simulink model "HODB"  (R2018b)
settings: Solver=FixedStepAuto  StartTime=0.0  StopTime=25  FixedStep=0.0025  RelTol=1e-3
settings Model: Creator=User  LastModifiedBy=User

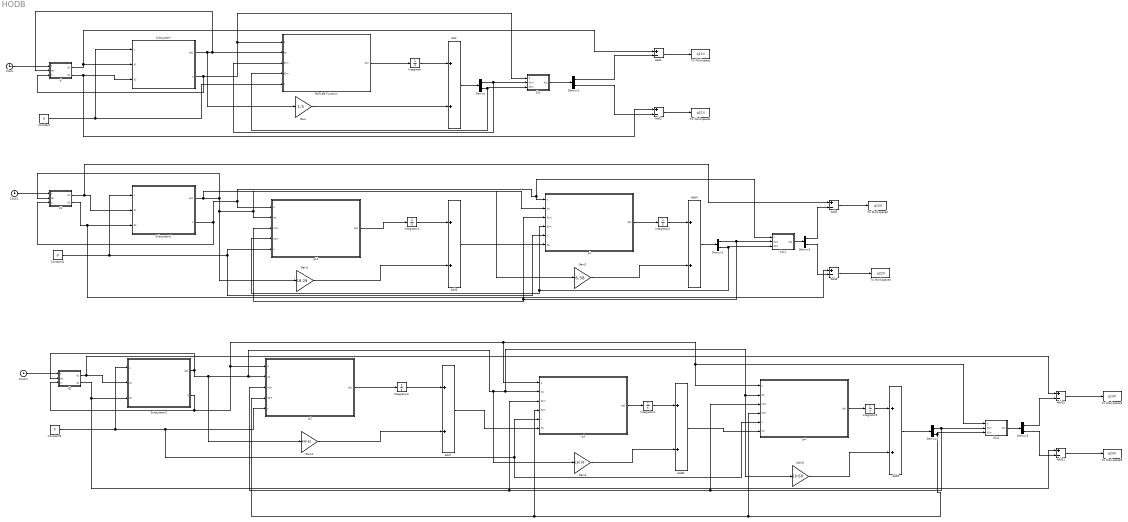
== system HODB ==
  Add{,3..4,7..9} (6 alike) : Sum
  Add{1..2,5..6,10..11} (6 alike) : Sum  Inputs=+-
  Clock : Clock
  Clock1 : Clock
  Clock2 : Clock
  Constant : Constant  Value=0
  Constant1 : Constant  Value=0
  Constant2 : Constant  Value=0
  Demux{,1..5} (6 alike) : Demux  Outputs=2
  Gain : Gain  Gain=1.5
  Gain1 : Gain  Gain=18.29
  Gain2 : Gain  Gain=6.58
  Gain3 : Gain  Gain=498.83
  Gain4 : Gain  Gain=156.99
  Gain5 : Gain  Gain=10.69
  Integrator{,1..5} (6 alike) : Integrator  InitialCondition=[0;0]
  MATLAB Function : MATLAB Function  TreatAsAtomicUnit=on
  Subsystem : Subsystem
  Subsystem1 : Subsystem
  Subsystem2 : Subsystem
  To Workspace : ToWorkspace  VariableName=q11II  SampleTime=-1
  To Workspace1 : ToWorkspace  VariableName=q21II  SampleTime=-1
  To Workspace2 : ToWorkspace  VariableName=q12II  SampleTime=-1
  To Workspace3 : ToWorkspace  VariableName=q22II  SampleTime=-1
  To Workspace4 : ToWorkspace  VariableName=q13II  SampleTime=-1
  To Workspace5 : ToWorkspace  VariableName=q23II  SampleTime=-1
  d : MATLAB Function  TreatAsAtomicUnit=on
  d1 : MATLAB Function  TreatAsAtomicUnit=on
  d1s : MATLAB Function  TreatAsAtomicUnit=on
  d1s1 : MATLAB Function  TreatAsAtomicUnit=on
  d1s2 : MATLAB Function  TreatAsAtomicUnit=on
  d2 : MATLAB Function  TreatAsAtomicUnit=on
  p1 : MATLAB Function  TreatAsAtomicUnit=on
  p12 : MATLAB Function  TreatAsAtomicUnit=on
  p2 : MATLAB Function  TreatAsAtomicUnit=on
  p3 : MATLAB Function  TreatAsAtomicUnit=on
  p4 : MATLAB Function  TreatAsAtomicUnit=on
  wires:
  MATLAB Function/1(dp1) -> Integrator/1
  Integrator/1 -> Add/1
  Subsystem/1(dq1) -> Gain/1, d/2(dq), MATLAB Function/2(dq)
  Subsystem/2(q) -> d/3(q), d1s/1(q), MATLAB Function/1(q)
  Gain/1 -> Add/2
  Add/1 -> Demux/1
  Demux/1 -> d1s/2(d1m), MATLAB Function/3(d1m)
  Demux/2 -> MATLAB Function/4(d2m), d1s/3(d2m)
  Constant/1 -> MATLAB Function/5(u), Subsystem/1(u)
  d/1(d1) -> Add1/1, Subsystem/2(d1)
  d/2(d2) -> Add2/1, Subsystem/3(d2)
  Clock/1 -> d/1(t)
  d1s/1(d1s) -> Demux1/1
  Demux1/1 -> Add1/2
  Demux1/2 -> Add2/2
  Add2/1 -> To Workspace1/1
  Add1/1 -> To Workspace/1
  Clock1/1 -> d1/1(t)
  Constant1/1 -> Subsystem1/1(u), p1/5(u), p12/5(u)
  d1/1(d1) -> Add5/1, Subsystem1/2(d1)
  d1/2(d2) -> Add6/1, Subsystem1/3(d2)
  Subsystem1/1(dq1) -> Gain2/1, Gain1/1, p1/2(dq), p12/2(dq), d1/2(dq)
  Subsystem1/2(q) -> d1s1/1(q), p1/1(q), p12/1(q), d1/3(q)
  p12/1(dp1) -> Integrator1/1
  Integrator1/1 -> Add3/1
  Gain1/1 -> Add3/2
  Add3/1 -> p1/6(d1i)
  p1/1(dp1) -> Integrator2/1
  Integrator2/1 -> Add4/1
  Gain2/1 -> Add4/2
  Add4/1 -> Demux2/1
  Demux2/1 -> d1s1/2(d1m), p1/3(d1m), p12/3(d1m)
  Demux2/2 -> d1s1/3(d2m), p1/4(d2m), p12/4(d2m)
  d1s1/1(d1s) -> Demux3/1
  Demux3/1 -> Add5/2
  Demux3/2 -> Add6/2
  Add5/1 -> To Workspace2/1
  Add6/1 -> To Workspace3/1
  d2/1(d1) -> Add10/1, Subsystem2/2(d1)
  d2/2(d2) -> Add11/1, Subsystem2/3(d2)
  Clock2/1 -> d2/1(t)
  Constant2/1 -> Subsystem2/1(u), p4/5(u), p3/5(u), p2/5(u)
  Subsystem2/1(dq1) -> Gain3/1, Gain4/1, Gain5/1, p4/2(dq), p3/2(dq), p2/2(dq), d2/2(dq)
  Subsystem2/2(q) -> p3/1(q), d1s2/1(q), p4/1(q), p2/1(q), d2/3(q)
  p2/1(dp1) -> Integrator3/1
  Integrator3/1 -> Add7/1
  Gain3/1 -> Add7/2
  Add7/1 -> p3/6(d1i)
  p3/1(dp1) -> Integrator4/1
  Gain4/1 -> Add8/2
  Add8/1 -> p4/6(d1i)
  p4/1(dp1) -> Integrator5/1
  Gain5/1 -> Add9/2
  Add9/1 -> Demux4/1
  Demux4/1 -> d1s2/2(d1m), p2/3(d1m), p3/3(d1m), p4/3(d1m)
  Demux4/2 -> d1s2/3(d2m), p2/4(d2m), p3/4(d2m), p4/4(d2m)
  d1s2/1(d1s) -> Demux5/1
  Demux5/1 -> Add10/2
  Demux5/2 -> Add11/2
  Add11/1 -> To Workspace5/1
  Add10/1 -> To Workspace4/1
  Integrator4/1 -> Add8/1
  Integrator5/1 -> Add9/1

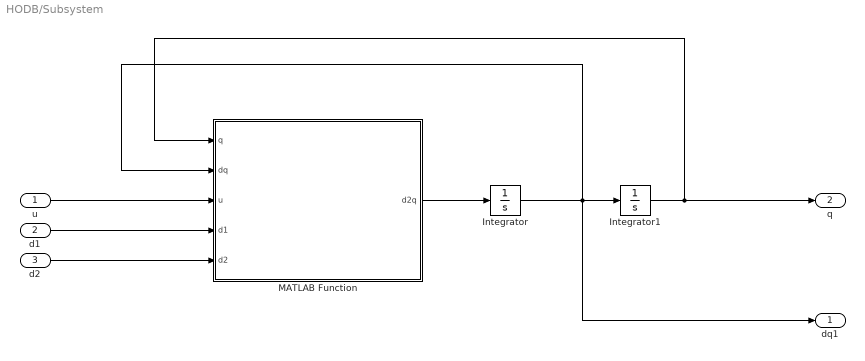
== system HODB/Subsystem ==
  u : Inport
  d1 : Inport  Port=2
  d2 : Inport  Port=3
  Integrator : Integrator  InitialCondition=[-0.01;0.05]
  Integrator1 : Integrator  InitialCondition=[-1.4208;-0.1]
  MATLAB Function : MATLAB Function  TreatAsAtomicUnit=on
  dq1 : Outport
  q : Outport  Port=2
  wires:
  Integrator1/1 -> q/1, MATLAB Function/1(q)
  d2/1 -> MATLAB Function/5(d2)
  d1/1 -> MATLAB Function/4(d1)
  Integrator/1 -> dq1/1, MATLAB Function/2(dq), Integrator1/1
  u/1 -> MATLAB Function/3(u)
  MATLAB Function/1(d2q) -> Integrator/1

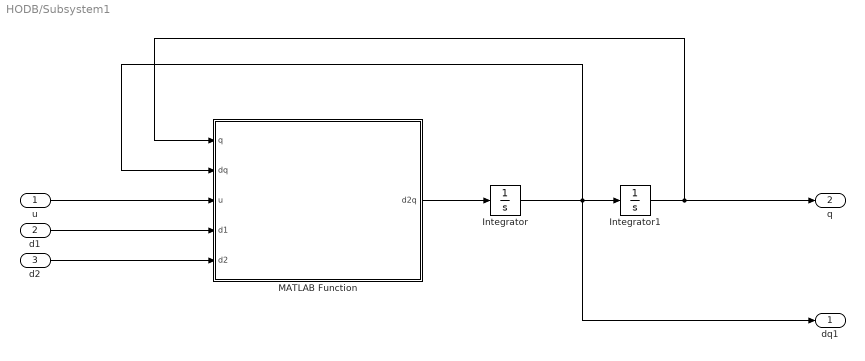
== system HODB/Subsystem1 ==
  u : Inport
  d1 : Inport  Port=2
  d2 : Inport  Port=3
  Integrator : Integrator  InitialCondition=[-0.01;0.05]
  Integrator1 : Integrator  InitialCondition=[-1.4208;-0.1]
  MATLAB Function : MATLAB Function  TreatAsAtomicUnit=on
  dq1 : Outport
  q : Outport  Port=2
  wires:
  MATLAB Function/1(d2q) -> Integrator/1
  u/1 -> MATLAB Function/3(u)
  Integrator/1 -> Integrator1/1, MATLAB Function/2(dq), dq1/1
  d1/1 -> MATLAB Function/4(d1)
  d2/1 -> MATLAB Function/5(d2)
  Integrator1/1 -> MATLAB Function/1(q), q/1

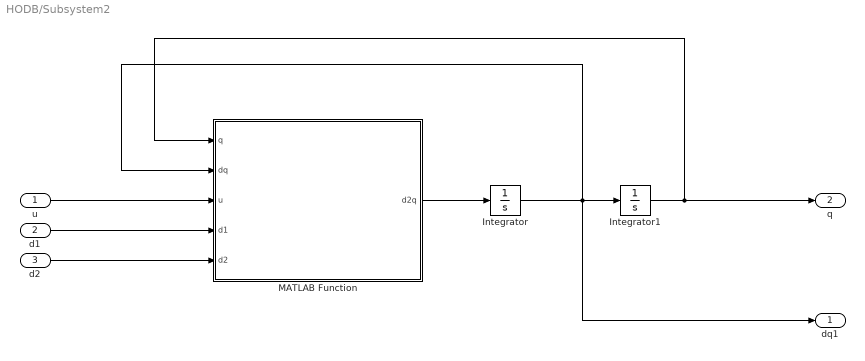
== system HODB/Subsystem2 ==
  u : Inport
  d1 : Inport  Port=2
  d2 : Inport  Port=3
  Integrator : Integrator  InitialCondition=[-0.01;0.05]
  Integrator1 : Integrator  InitialCondition=[-1.4208;-0.1]
  MATLAB Function : MATLAB Function  TreatAsAtomicUnit=on
  dq1 : Outport
  q : Outport  Port=2
  wires:
  Integrator1/1 -> q/1, MATLAB Function/1(q)
  d2/1 -> MATLAB Function/5(d2)
  d1/1 -> MATLAB Function/4(d1)
  Integrator/1 -> dq1/1, MATLAB Function/2(dq), Integrator1/1
  u/1 -> MATLAB Function/3(u)
  MATLAB Function/1(d2q) -> Integrator/1

== matlab function HODB/MATLAB Function ==
  data: q input; dq input; d1m input; d2m input; u input; dp1 output
function dp1 = fcn(q,dq,d1m,d2m,u)
L1=1.5;
m1=1;
m2=1;
l1=1;
% l2=2;
lc1=0.5;
lc2=1;
I1=0.083;
I2=0.33;
a0=m1*lc1^2+m2*(l1^2+lc2^2)+I1+I2;
b0=2*m2*l1*lc2;
c0=m2*lc2^2+I2;
q1=q(1);
q2=q(2);
m11=a0+b0*cos(q2);
m12=c0+0.5*b0*cos(q2);
m21=m12;
m22=c0;
M=[m11 m12;m21 m22];
g=9.81;
dq1=dq(1);
dq2=dq(2);
h1=-m2*l1*lc2*sin(q2)*dq2^2-2*m2*l1*lc2*sin(q2)*dq1*dq2;
h2=m2*l1*lc2*sin(q2)*dq1^2;
phi1=(m1*lc1+m2*l1)*g*cos(q1)+m2*lc2*g*cos(q1+q2);
phi2=m2*lc2*g*cos(q1+q2);
dp1=-L1*(-M\[h1+phi1;h2+phi2]+[d1m;d2m]+M\[0;u]);
end

== matlab function HODB/Subsystem/MATLAB Function ==
  data: q input; dq input; u input; d2q output; d1 input; d2 input
function d2q = fcn(q,dq,u,d1,d2)
m1=1;
m2=1;
l1=1;
% l2=2;
lc1=0.5;
lc2=1;
I1=0.083;
I2=0.33;
a0=m1*lc1^2+m2*(l1^2+lc2^2)+I1+I2;
b0=2*m2*l1*lc2;
c0=m2*lc2^2+I2;
q1=q(1);
q2=q(2);
m11=a0+b0*cos(q2);
m12=c0+0.5*b0*cos(q2);
m21=m12;
m22=c0;
g=9.81;
dq1=dq(1);
dq2=dq(2);
h1=-m2*l1*lc2*sin(q2)*dq2^2-2*m2*l1*lc2*sin(q2)*dq1*dq2;
h2=m2*l1*lc2*sin(q2)*dq1^2;
phi1=(m1*lc1+m2*l1)*g*cos(q1)+m2*lc2*g*cos(q1+q2);
phi2=m2*lc2*g*cos(q1+q2);
d2q=[m11 m12;m21 m22]\[d1-h1-phi1;u+d2-h2-phi2];
end

== matlab function HODB/d ==
  data: t input; d1 output; dq input; q input; d2 output
function [d1,d2] = fcn(t,dq,q)
d1=0.1*sin(t+pi/2)+0.04*sin(5.3*t)-0.05*dq(1)+0.01*q(1);
d2=0.1*sin(t*2)+0.02*sin(4.6*t+0.5)-0.03*dq(2)+0.008*q(2);
% d1=0.1*sin(t+pi/2)+0.04*sin(5.3*t);
% d2=0.1*sin(t*2)+0.02*sin(4.6*t+0.5);
% d1=0.05;
% d2=0.03;
end

== matlab function HODB/d1s ==
  data: q input; d1s output; d1m input; d2m input
function d1s = fcn(q,d1m,d2m)
m1=1;
m2=1;
l1=1;
% l2=2;
lc1=0.5;
lc2=1;
I1=0.083;
I2=0.33;
a0=m1*lc1^2+m2*(l1^2+lc2^2)+I1+I2;
b0=2*m2*l1*lc2;
c0=m2*lc2^2+I2;
% q1=q(1);
q2=q(2);
m11=a0+b0*cos(q2);
m12=c0+0.5*b0*cos(q2);
m21=m12;
m22=c0;
M=[m11 m12;m21 m22];
d1s=M*[d1m;d2m];
end

== matlab function HODB/Subsystem1/MATLAB Function ==
  data: q input; dq input; u input; d2q output; d1 input; d2 input
function d2q = fcn(q,dq,u,d1,d2)
m1=1;
m2=1;
l1=1;
% l2=2;
lc1=0.5;
lc2=1;
I1=0.083;
I2=0.33;
a0=m1*lc1^2+m2*(l1^2+lc2^2)+I1+I2;
b0=2*m2*l1*lc2;
c0=m2*lc2^2+I2;
q1=q(1);
q2=q(2);
m11=a0+b0*cos(q2);
m12=c0+0.5*b0*cos(q2);
m21=m12;
m22=c0;
g=9.81;
dq1=dq(1);
dq2=dq(2);
h1=-m2*l1*lc2*sin(q2)*dq2^2-2*m2*l1*lc2*sin(q2)*dq1*dq2;
h2=m2*l1*lc2*sin(q2)*dq1^2;
phi1=(m1*lc1+m2*l1)*g*cos(q1)+m2*lc2*g*cos(q1+q2);
phi2=m2*lc2*g*cos(q1+q2);
d2q=[m11 m12;m21 m22]\[d1-h1-phi1;u+d2-h2-phi2];
end

== matlab function HODB/d1 ==
  data: t input; d1 output; dq input; q input; d2 output
function [d1,d2] = fcn(t,dq,q)
d1=0.1*sin(t+pi/2)+0.04*sin(5.3*t)-0.05*dq(1)+0.01*q(1);
d2=0.1*sin(t*2)+0.02*sin(4.6*t+0.5)-0.03*dq(2)+0.008*q(2);
% d1=0.1*sin(t+pi/2)+0.04*sin(5.3*t);
% d2=0.1*sin(t*2)+0.02*sin(4.6*t+0.5);
% d1=0.05;
% d2=0.03;
end

== matlab function HODB/p12 ==
  data: q input; dq input; d1m input; d2m input; u input; dp1 output
function dp1 = fcn(q,dq,d1m,d2m,u)
L1=18.29;
m1=1;
m2=1;
l1=1;
% l2=2;
lc1=0.5;
lc2=1;
I1=0.083;
I2=0.33;
a0=m1*lc1^2+m2*(l1^2+lc2^2)+I1+I2;
b0=2*m2*l1*lc2;
c0=m2*lc2^2+I2;
q1=q(1);
q2=q(2);
m11=a0+b0*cos(q2);
m12=c0+0.5*b0*cos(q2);
m21=m12;
m22=c0;
M=[m11 m12;m21 m22];
g=9.81;
dq1=dq(1);
dq2=dq(2);
h1=-m2*l1*lc2*sin(q2)*dq2^2-2*m2*l1*lc2*sin(q2)*dq1*dq2;
h2=m2*l1*lc2*sin(q2)*dq1^2;
phi1=(m1*lc1+m2*l1)*g*cos(q1)+m2*lc2*g*cos(q1+q2);
phi2=m2*lc2*g*cos(q1+q2);
dp1=-L1*(-M\[h1+phi1;h2+phi2]+[d1m;d2m]+M\[0;u]);
end

== matlab function HODB/p1 ==
  data: q input; dq input; d1m input; d2m input; u input; dp1 output; d1i input
function dp1 = fcn(q,dq,d1m,d2m,u,d1i)
L1=6.58;
m1=1;
m2=1;
l1=1;
% l2=2;
lc1=0.5;
lc2=1;
I1=0.083;
I2=0.33;
a0=m1*lc1^2+m2*(l1^2+lc2^2)+I1+I2;
b0=2*m2*l1*lc2;
c0=m2*lc2^2+I2;
q1=q(1);
q2=q(2);
m11=a0+b0*cos(q2);
m12=c0+0.5*b0*cos(q2);
m21=m12;
m22=c0;
M=[m11 m12;m21 m22];
g=9.81;
dq1=dq(1);
dq2=dq(2);
h1=-m2*l1*lc2*sin(q2)*dq2^2-2*m2*l1*lc2*sin(q2)*dq1*dq2;
h2=m2*l1*lc2*sin(q2)*dq1^2;
phi1=(m1*lc1+m2*l1)*g*cos(q1)+m2*lc2*g*cos(q1+q2);
phi2=m2*lc2*g*cos(q1+q2);
dp1=-L1*(-M\[h1+phi1;h2+phi2]+[d1m;d2m]+M\[0;u])+d1i;
end

== matlab function HODB/d1s1 ==
  data: q input; d1s output; d1m input; d2m input
function d1s = fcn(q,d1m,d2m)
m1=1;
m2=1;
l1=1;
% l2=2;
lc1=0.5;
lc2=1;
I1=0.083;
I2=0.33;
a0=m1*lc1^2+m2*(l1^2+lc2^2)+I1+I2;
b0=2*m2*l1*lc2;
c0=m2*lc2^2+I2;
% q1=q(1);
q2=q(2);
m11=a0+b0*cos(q2);
m12=c0+0.5*b0*cos(q2);
m21=m12;
m22=c0;
M=[m11 m12;m21 m22];
d1s=M*[d1m;d2m];
end

== matlab function HODB/p3 ==
  data: q input; dq input; d1m input; d2m input; u input; dp1 output; d1i input
function dp1 = fcn(q,dq,d1m,d2m,u,d1i)
L1=156.99;
m1=1;
m2=1;
l1=1;
% l2=2;
lc1=0.5;
lc2=1;
I1=0.083;
I2=0.33;
a0=m1*lc1^2+m2*(l1^2+lc2^2)+I1+I2;
b0=2*m2*l1*lc2;
c0=m2*lc2^2+I2;
q1=q(1);
q2=q(2);
m11=a0+b0*cos(q2);
m12=c0+0.5*b0*cos(q2);
m21=m12;
m22=c0;
M=[m11 m12;m21 m22];
g=9.81;
dq1=dq(1);
dq2=dq(2);
h1=-m2*l1*lc2*sin(q2)*dq2^2-2*m2*l1*lc2*sin(q2)*dq1*dq2;
h2=m2*l1*lc2*sin(q2)*dq1^2;
phi1=(m1*lc1+m2*l1)*g*cos(q1)+m2*lc2*g*cos(q1+q2);
phi2=m2*lc2*g*cos(q1+q2);
dp1=-L1*(-M\[h1+phi1;h2+phi2]+[d1m;d2m]+M\[0;u])+d1i;
end

== matlab function HODB/Subsystem2/MATLAB Function ==
  data: q input; dq input; u input; d2q output; d1 input; d2 input
function d2q = fcn(q,dq,u,d1,d2)
m1=1;
m2=1;
l1=1;
% l2=2;
lc1=0.5;
lc2=1;
I1=0.083;
I2=0.33;
a0=m1*lc1^2+m2*(l1^2+lc2^2)+I1+I2;
b0=2*m2*l1*lc2;
c0=m2*lc2^2+I2;
q1=q(1);
q2=q(2);
m11=a0+b0*cos(q2);
m12=c0+0.5*b0*cos(q2);
m21=m12;
m22=c0;
g=9.81;
dq1=dq(1);
dq2=dq(2);
h1=-m2*l1*lc2*sin(q2)*dq2^2-2*m2*l1*lc2*sin(q2)*dq1*dq2;
h2=m2*l1*lc2*sin(q2)*dq1^2;
phi1=(m1*lc1+m2*l1)*g*cos(q1)+m2*lc2*g*cos(q1+q2);
phi2=m2*lc2*g*cos(q1+q2);
d2q=[m11 m12;m21 m22]\[d1-h1-phi1;u+d2-h2-phi2];
end

== matlab function HODB/d2 ==
  data: t input; d1 output; dq input; q input; d2 output
function [d1,d2] = fcn(t,dq,q)
d1=0.1*sin(t+pi/2)+0.04*sin(5.3*t)-0.05*dq(1)+0.01*q(1);
d2=0.1*sin(t*2)+0.02*sin(4.6*t+0.5)-0.03*dq(2)+0.008*q(2);
% d1=0.1*sin(t+pi/2)+0.04*sin(5.3*t);
% d2=0.1*sin(t*2)+0.02*sin(4.6*t+0.5);
% d1=0.05;
% d2=0.03;
end

== matlab function HODB/p2 ==
  data: q input; dq input; d1m input; d2m input; u input; dp1 output
function dp1 = fcn(q,dq,d1m,d2m,u)
L1=498.83;
m1=1;
m2=1;
l1=1;
% l2=2;
lc1=0.5;
lc2=1;
I1=0.083;
I2=0.33;
a0=m1*lc1^2+m2*(l1^2+lc2^2)+I1+I2;
b0=2*m2*l1*lc2;
c0=m2*lc2^2+I2;
q1=q(1);
q2=q(2);
m11=a0+b0*cos(q2);
m12=c0+0.5*b0*cos(q2);
m21=m12;
m22=c0;
M=[m11 m12;m21 m22];
g=9.81;
dq1=dq(1);
dq2=dq(2);
h1=-m2*l1*lc2*sin(q2)*dq2^2-2*m2*l1*lc2*sin(q2)*dq1*dq2;
h2=m2*l1*lc2*sin(q2)*dq1^2;
phi1=(m1*lc1+m2*l1)*g*cos(q1)+m2*lc2*g*cos(q1+q2);
phi2=m2*lc2*g*cos(q1+q2);
dp1=-L1*(-M\[h1+phi1;h2+phi2]+[d1m;d2m]+M\[0;u]);
end

== matlab function HODB/p4 ==
  data: q input; dq input; d1m input; d2m input; u input; dp1 output; d1i input
function dp1 = fcn(q,dq,d1m,d2m,u,d1i)
L1=10.69;
m1=1;
m2=1;
l1=1;
% l2=2;
lc1=0.5;
lc2=1;
I1=0.083;
I2=0.33;
a0=m1*lc1^2+m2*(l1^2+lc2^2)+I1+I2;
b0=2*m2*l1*lc2;
c0=m2*lc2^2+I2;
q1=q(1);
q2=q(2);
m11=a0+b0*cos(q2);
m12=c0+0.5*b0*cos(q2);
m21=m12;
m22=c0;
M=[m11 m12;m21 m22];
g=9.81;
dq1=dq(1);
dq2=dq(2);
h1=-m2*l1*lc2*sin(q2)*dq2^2-2*m2*l1*lc2*sin(q2)*dq1*dq2;
h2=m2*l1*lc2*sin(q2)*dq1^2;
phi1=(m1*lc1+m2*l1)*g*cos(q1)+m2*lc2*g*cos(q1+q2);
phi2=m2*lc2*g*cos(q1+q2);
dp1=-L1*(-M\[h1+phi1;h2+phi2]+[d1m;d2m]+M\[0;u])+d1i;
end

== matlab function HODB/d1s2 ==
  data: q input; d1s output; d1m input; d2m input
function d1s = fcn(q,d1m,d2m)
m1=1;
m2=1;
l1=1;
% l2=2;
lc1=0.5;
lc2=1;
I1=0.083;
I2=0.33;
a0=m1*lc1^2+m2*(l1^2+lc2^2)+I1+I2;
b0=2*m2*l1*lc2;
c0=m2*lc2^2+I2;
% q1=q(1);
q2=q(2);
m11=a0+b0*cos(q2);
m12=c0+0.5*b0*cos(q2);
m21=m12;
m22=c0;
M=[m11 m12;m21 m22];
d1s=M*[d1m;d2m];
end
